simulink model "AB_Final_of_MPC_Bandwidth_Result_UnbalancedNew"  (R2022b)
settings: Solver=FixedStepDiscrete  StartTime=0.0  StopTime=Inf  FixedStep=100e-6  RelTol=1e-3  EnableMultiTasking=on
undefined symbols (not defined in the file): C28x, CPU1, CPU2, CurrentBypassValue, DiscIntNeverNeededParam, Down, GPTRIP1SEL, TZ1, Up
libraries: c2802xlib x20, simulink x17, dspstat3 x13, eeGeneralControl x10, c2837xDlib x5, c280xlib x5, PID_Lib x4, c2000lib x1, spsAlphaBetaZerotoabcLib x1
(part 9 of 10)

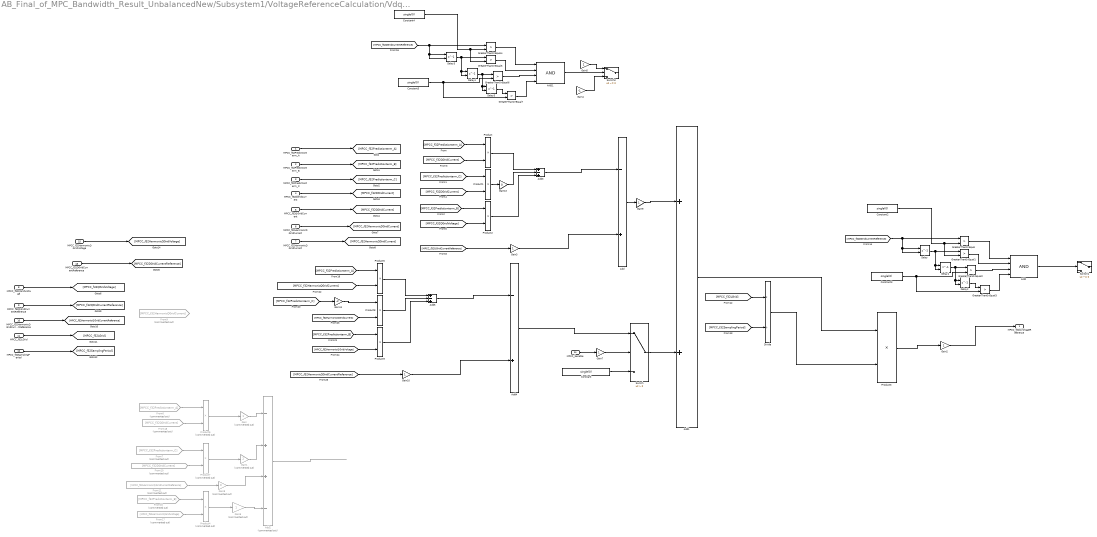
== system AB_Final_of_MPC_Bandwidth_Result_UnbalancedNew/Subsystem1/VoltageReferenceCalculation/VdqVoltageReferenceCalculation/VqVoltageReferenceCalculation ==
  MPCC_f32Predictionterm_A : Inport
  MPCC_f32Predictionterm_B : Inport  Port=2
  MPCC_f32Predictionterm_C : Inport  Port=3
  MPCC_f32DGridCurrent : Inport  Port=4
  MPCC_f32QGridCurrent : Inport  Port=5
  MPCC_f32HarmonicDGridCurrent : Inport  Port=6
  MPCC_f32HarmonicQGridCurrent : Inport  Port=7
  MPCC_f32QGridVoltage : Inport  Port=8
  MPCC_f32QGridCurrentReference : Inport  Port=9
  MPCC_f32HarmonicQGridCurrentReference : Inport  Port=10
  MPCC_f32LGrid : Inport  Port=11
  MPCC_f32SamplingPeriod : Inport  Port=12
  MPCC_f32DGridCurrentReference : Inport  Port=13
  MPCC_benable : Inport  Port=14
  MPCC_f32HarmonicQGridVoltage : Inport  Port=15
  AND : Logic  Inputs=4  AllPortsSameDT=off  OutDataTypeStr=boolean
  AND1 : Logic  Inputs=4  AllPortsSameDT=off  OutDataTypeStr=boolean
  Add : Sum  Inputs=-+
  Add1 : Sum
  Add2 : Sum  Commented=on  Inputs=-++-
  Add3 : Sum  Inputs=+-+
  Add4 : Sum  Inputs=-+
  Add5 : Sum  Inputs=+-+
  Constant{,2..5} (5 alike) : Constant  Value=single(0)
  Delay{,1..5} (6 alike) : Delay  DelayLength=1  InitialConditionSource=Input port
      settings: InputPortMap=u0,p4
  Divide : Product  Inputs=*/  RndMeth=Zero  SaturateOnIntegerOverflow=on
  From10 : From  Commented=on  GotoTag=MPCC_f32DGridCurrent
  From11 : From  Commented=on  GotoTag=MPCC_f32HarmonicQGridCurrentReference
  From15 : From  Commented=on  GotoTag=MPCC_f32Predictionterm_B
  From17 : From  Commented=on  GotoTag=MPCC_f32HarmonicQGridVoltage
  From18 : From  Commented=on  GotoTag=MPCC_f32QGridCurrent
  From6 : From  Commented=on  GotoTag=MPCC_f32Predictionterm_A
  From7 : From  Commented=on  GotoTag=MPCC_f32Predictionterm_C
  From9 : From  Commented=on  GotoTag=MPCC_f32HarmonicQGridCurrent
  Gain : Gain  Commented=on
  Gain1 : Gain  Commented=on  Gain=2
  Gain{2..3,5,7,9..10} (6 alike) : Gain
  Gain11 : Gain  Gain=-2
  Gain13 : Gain  Gain=0
  Gain4 : Gain  Gain=-1
  Gain6 : Gain  Commented=on
  Gain8 : Gain  Commented=on  Gain=0
  GreaterThanOrEqual{,1..7} (8 alike) : RelationalOperator  Operator=>  OutDataTypeStr=boolean  RndMeth=Simplest  InputSameDT=off
  Product{,1..3,5,8..9} (7 alike) : Product
  Product4 : Product  Commented=on
  Product6 : Product  Commented=on
  Product7 : Product  Commented=on
  Switch : Switch  Criteria=u2 > Threshold  SaturateOnIntegerOverflow=off  InputSameDT=off
  Switch1 : Switch  Criteria=u2 ~= 0  SaturateOnIntegerOverflow=off  InputSameDT=off
  Switch2 : Switch  Criteria=u2 ~= 0  SaturateOnIntegerOverflow=off  InputSameDT=off
  MPCC_f32QVoltageReference : Outport
  wires:
  [MPCC_f32DGridCurrent] -> Product1/2
  [MPCC_f32Predictionterm_A] -> Product/1
  [MPCC_f32QGridVoltage] -> Product2/2
  [MPCC_f32QGridCurrent] -> Product/2
  [MPCC_f32Predictionterm_C] -> Product1/1
  [MPCC_f32Predictionterm_B] -> Product2/1
  MPCC_f32Predictionterm_A/1 -> [MPCC_f32Predictionterm_A]
  MPCC_f32Predictionterm_B/1 -> [MPCC_f32Predictionterm_B]
  MPCC_f32Predictionterm_C/1 -> [MPCC_f32Predictionterm_C]
  MPCC_f32DGridCurrent/1 -> [MPCC_f32DGridCurrent]
  MPCC_f32QGridCurrent/1 -> [MPCC_f32QGridCurrent]
  MPCC_f32HarmonicDGridCurrent/1 -> [MPCC_f32HarmonicDGridCurrent]
  MPCC_f32HarmonicQGridCurrent/1 -> [MPCC_f32HarmonicQGridCurrent]
  MPCC_f32QGridVoltage/1 -> [MPCC_f32QGridVoltage]
  Constant/1 -> Switch/3
  MPCC_benable/1 -> Gain7/1
  Switch/1 -> Add1/2
  Add/1 -> Gain9/1
  MPCC_f32QGridCurrentReference/1 -> [MPCC_f32QGridCurrentReference]
  MPCC_f32HarmonicQGridCurrentReference/1 -> [MPCC_f32HarmonicQGridCurrentReference]
  [MPCC_f32QGridCurrentReference] -> Gain3/1
  MPCC_f32LGrid/1 -> [MPCC_f32LGrid]
  MPCC_f32SamplingPeriod/1 -> [MPCC_f32SamplingPeriod]
  [MPCC_f32LGrid] -> Divide/1
  [MPCC_f32SamplingPeriod] -> Divide/2
  MPCC_f32DGridCurrentReference/1 -> [MPCC_f32DGridCurrentReference]
  Gain2/1 -> MPCC_f32QVoltageReference/1
  GreaterThanOrEqual2/1 -> AND/3
  Constant3/1 -> GreaterThanOrEqual3/2, GreaterThanOrEqual2/2
  Constant2/1 -> GreaterThanOrEqual1/2, GreaterThanOrEqual/2
  Delay2/1 -> GreaterThanOrEqual3/1
  GreaterThanOrEqual1/1 -> AND/2
  Delay/1 -> GreaterThanOrEqual1/1, Delay1/2, Delay1/1
  Divide/1 -> Product3/2
  GreaterThanOrEqual/1 -> AND/1
  GreaterThanOrEqual3/1 -> AND/4
  Delay1/1 -> Delay2/2, Delay2/1, GreaterThanOrEqual2/1
  [MPCC_f32DGridCurrentReference] -> GreaterThanOrEqual/1, Delay/2, Delay/1
  Product3/1 -> Gain2/1
  AND/1 -> Switch1/2
  Product/1 -> Add3/1
  Product1/1 -> Gain13/1
  Product2/1 -> Add3/3
  Gain3/1 -> Add/2
  AND1/1 -> Switch2/2
  GreaterThanOrEqual7/1 -> AND1/4
  GreaterThanOrEqual6/1 -> AND1/3
  Delay5/1 -> GreaterThanOrEqual7/1
  GreaterThanOrEqual4/1 -> AND1/1
  Delay3/1 -> GreaterThanOrEqual5/1, Delay4/2, Delay4/1
  GreaterThanOrEqual5/1 -> AND1/2
  Constant5/1 -> GreaterThanOrEqual7/2, GreaterThanOrEqual6/2
  Delay4/1 -> Delay5/2, Delay5/1, GreaterThanOrEqual6/1
  Constant4/1 -> GreaterThanOrEqual5/2, GreaterThanOrEqual4/2
  [MPCC_f32DGridCurrentReference] -> GreaterThanOrEqual4/1, Delay3/2, Delay3/1
  Gain5/1 -> Switch2/1
  Gain4/1 -> Switch2/3
  Add1/1 -> Product3/1
  Add3/1 -> Add/1
  MPCC_f32HarmonicQGridVoltage/1 -> [MPCC_f32HarmonicQGridVoltage]
  Gain7/1 -> Switch/2
  Gain9/1 -> Add1/1
  Gain/1 -> Add2/1
  From6/1 -> Product6/1
  From11/1 -> Gain8/1
  From18/1 -> Product6/2
  From10/1 -> Product7/2
  Product7/1 -> Gain1/1
  Gain6/1 -> Add2/4
  Product6/1 -> Gain/1
  Add2/1 -> ?
  Product4/1 -> Gain6/1
  From15/1 -> Product4/1
  Gain8/1 -> Add2/3
  From7/1 -> Product7/1
  Gain1/1 -> Add2/2
  From17/1 -> Product4/2
  [MPCC_f32Predictionterm_B] -> Product9/1
  [MPCC_f32Predictionterm_C] -> Gain11/1
  [MPCC_f32HarmonicDGridCurrent] -> Product8/2
  [MPCC_f32HarmonicQGridCurrentReference] -> Gain10/1
  Add5/1 -> Add4/1
  Product5/1 -> Add5/1
  [MPCC_f32Predictionterm_A] -> Product5/1
  Gain10/1 -> Add4/2
  Product8/1 -> Add5/2
  Product9/1 -> Add5/3
  [MPCC_f32HarmonicQGridVoltage] -> Product9/2
  [MPCC_f32HarmonicQGridCurrent] -> Product5/2
  Add4/1 -> Switch/1
  Gain11/1 -> Product8/1
  Gain13/1 -> Add3/2

== system AB_Final_of_MPC_Bandwidth_Result_UnbalancedNew/Subsystem3/PLL_Loop2/SOGI 1st3/Integrator ==
  In : Inport
  Delay1 : Delay  DelayLength=1
  Delay2 : Delay  DelayLength=1
  Delay3 : Delay  DelayLength=1
  Gain : Gain  Gain=100e-6/12
  Gain1 : Gain  Gain=23
  Gain2 : Gain  Gain=16
  Gain3 : Gain  Gain=5
  Sum : Sum  Inputs=|+-
  Sum1 : Sum  Inputs=|++
  Sum2 : Sum  Inputs=|++
  Out : Outport
  wires:
  Delay2/1 -> Gain2/1, Delay3/1
  Delay1/1 -> Sum2/2, Gain1/1, Delay2/1
  Delay3/1 -> Gain3/1
  Gain2/1 -> Sum/2
  Gain1/1 -> Sum/1
  Gain3/1 -> Sum1/2
  Sum/1 -> Sum1/1
  Gain/1 -> Sum2/1
  Sum2/1 -> Delay1/1
  In/1 -> Gain/1
  Sum1/1 -> Out/1

== system AB_Final_of_MPC_Bandwidth_Result_UnbalancedNew/Subsystem3/PLL_Loop2/SOGI 1st3/Integrator1 ==
  In : Inport
  Delay1 : Delay  DelayLength=1
  Delay2 : Delay  DelayLength=1
  Delay3 : Delay  DelayLength=1
  Gain : Gain  Gain=100e-6/12
  Gain1 : Gain  Gain=23
  Gain2 : Gain  Gain=16
  Gain3 : Gain  Gain=5
  Sum : Sum  Inputs=|+-
  Sum1 : Sum  Inputs=|++
  Sum2 : Sum  Inputs=|++
  Out : Outport
  wires:
  Delay2/1 -> Gain2/1, Delay3/1
  Delay1/1 -> Sum2/2, Gain1/1, Delay2/1
  Delay3/1 -> Gain3/1
  Gain2/1 -> Sum/2
  Gain1/1 -> Sum/1
  Gain3/1 -> Sum1/2
  Sum/1 -> Sum1/1
  Gain/1 -> Sum2/1
  Sum2/1 -> Delay1/1
  In/1 -> Gain/1
  Sum1/1 -> Out/1

== system AB_Final_of_MPC_Bandwidth_Result_UnbalancedNew/Subsystem3/PLL_Loop2/SOGI 1st3/Integrator2 ==
  In : Inport
  Delay1 : Delay  DelayLength=1
  Delay2 : Delay  DelayLength=1
  Delay3 : Delay  DelayLength=1
  Gain : Gain  Gain=100e-6/12
  Gain1 : Gain  Gain=23
  Gain2 : Gain  Gain=16
  Gain3 : Gain  Gain=5
  Sum : Sum  Inputs=|+-
  Sum1 : Sum  Inputs=|++
  Sum2 : Sum  Inputs=|++
  Out : Outport
  wires:
  In/1 -> Gain/1
  Delay2/1 -> Gain2/1, Delay3/1
  Delay1/1 -> Sum2/2, Gain1/1, Delay2/1
  Delay3/1 -> Gain3/1
  Gain2/1 -> Sum/2
  Gain1/1 -> Sum/1
  Gain3/1 -> Sum1/2
  Sum/1 -> Sum1/1
  Sum1/1 -> Out/1
  Gain/1 -> Sum2/1
  Sum2/1 -> Delay1/1

== system AB_Final_of_MPC_Bandwidth_Result_UnbalancedNew/Subsystem3/PLL_Loop2/SOGI 1st5/Integrator ==
  In : Inport
  Delay1 : Delay  DelayLength=1
  Delay2 : Delay  DelayLength=1
  Delay3 : Delay  DelayLength=1
  Gain : Gain  Gain=100e-6/12
  Gain1 : Gain  Gain=23
  Gain2 : Gain  Gain=16
  Gain3 : Gain  Gain=5
  Sum : Sum  Inputs=|+-
  Sum1 : Sum  Inputs=|++
  Sum2 : Sum  Inputs=|++
  Out : Outport
  wires:
  Delay2/1 -> Gain2/1, Delay3/1
  Delay1/1 -> Sum2/2, Gain1/1, Delay2/1
  Delay3/1 -> Gain3/1
  Gain2/1 -> Sum/2
  Gain1/1 -> Sum/1
  Gain3/1 -> Sum1/2
  Sum/1 -> Sum1/1
  Gain/1 -> Sum2/1
  Sum2/1 -> Delay1/1
  In/1 -> Gain/1
  Sum1/1 -> Out/1

== system AB_Final_of_MPC_Bandwidth_Result_UnbalancedNew/Subsystem3/PLL_Loop2/SOGI 1st5/Integrator1 ==
  In : Inport
  Delay1 : Delay  DelayLength=1
  Delay2 : Delay  DelayLength=1
  Delay3 : Delay  DelayLength=1
  Gain : Gain  Gain=100e-6/12
  Gain1 : Gain  Gain=23
  Gain2 : Gain  Gain=16
  Gain3 : Gain  Gain=5
  Sum : Sum  Inputs=|+-
  Sum1 : Sum  Inputs=|++
  Sum2 : Sum  Inputs=|++
  Out : Outport
  wires:
  Delay2/1 -> Gain2/1, Delay3/1
  Delay1/1 -> Sum2/2, Gain1/1, Delay2/1
  Delay3/1 -> Gain3/1
  Gain2/1 -> Sum/2
  Gain1/1 -> Sum/1
  Gain3/1 -> Sum1/2
  Sum/1 -> Sum1/1
  Gain/1 -> Sum2/1
  Sum2/1 -> Delay1/1
  In/1 -> Gain/1
  Sum1/1 -> Out/1

== system AB_Final_of_MPC_Bandwidth_Result_UnbalancedNew/Subsystem3/PLL_Loop2/SOGI 1st5/Integrator2 ==
  In : Inport
  Delay1 : Delay  DelayLength=1
  Delay2 : Delay  DelayLength=1
  Delay3 : Delay  DelayLength=1
  Gain : Gain  Gain=100e-6/12
  Gain1 : Gain  Gain=23
  Gain2 : Gain  Gain=16
  Gain3 : Gain  Gain=5
  Sum : Sum  Inputs=|+-
  Sum1 : Sum  Inputs=|++
  Sum2 : Sum  Inputs=|++
  Out : Outport
  wires:
  In/1 -> Gain/1
  Delay2/1 -> Gain2/1, Delay3/1
  Delay1/1 -> Sum2/2, Gain1/1, Delay2/1
  Delay3/1 -> Gain3/1
  Gain2/1 -> Sum/2
  Gain1/1 -> Sum/1
  Gain3/1 -> Sum1/2
  Sum/1 -> Sum1/1
  Sum1/1 -> Out/1
  Gain/1 -> Sum2/1
  Sum2/1 -> Delay1/1

== system AB_Final_of_MPC_Bandwidth_Result_UnbalancedNew/Subsystem1/AlphaBetaDutiesCalculation/DutiesCalculation/Duty_Sector1/DutyA_Sector1 ==
  MPCC_f32AlphaVoltageReference : Inport
  MPCC_f32BetaVoltageReference : Inport  Port=2
  MPCC_f32AlphaConvVoltage1 : Inport  Port=3
  MPCC_f32AlphaConvVoltage2 : Inport  Port=4
  MPCC_f32BetaConvVoltage1 : Inport  Port=5
  MPCC_f32BetaConvVoltage2 : Inport  Port=6
  Add : Sum  Inputs=+-
  Add1 : Sum  Inputs=+-
  Data Type Conversion : DataTypeConversion  OutDataTypeStr=single  SaturateOnIntegerOverflow=off  RndMeth=Floor
  Divide : Product  Inputs=*/  RndMeth=Zero  SaturateOnIntegerOverflow=on
  Product{,1..3} (4 alike) : Product
  MPCC_f32DutyA_Sector1 : Outport
  wires:
  [MPCC_f32AlphaVoltageReference] -> Product1/1
  Divide/1 -> Data Type Conversion/1
  [MPCC_f32AlphaConvVoltage2] -> Product/2
  [MPCC_f32AlphaConvVoltage1] -> Product3/1
  Add/1 -> Divide/1
  [MPCC_f32BetaConvVoltage2] -> Product1/2
  Product/1 -> Add/1
  Add1/1 -> Divide/2
  Product2/1 -> Add1/1
  [MPCC_f32BetaConvVoltage1] -> Product2/2
  [MPCC_f32AlphaConvVoltage2] -> Product2/1
  Product3/1 -> Add1/2
  [MPCC_f32BetaConvVoltage2] -> Product3/2
  Product1/1 -> Add/2
  MPCC_f32BetaConvVoltage1/1 -> [MPCC_f32BetaConvVoltage1]
  MPCC_f32AlphaVoltageReference/1 -> [MPCC_f32AlphaVoltageReference]
  MPCC_f32AlphaConvVoltage2/1 -> [MPCC_f32AlphaConvVoltage2]
  MPCC_f32BetaVoltageReference/1 -> [MPCC_f32BetaVoltageReference]
  MPCC_f32AlphaConvVoltage1/1 -> [MPCC_f32AlphaConvVoltage1]
  MPCC_f32BetaConvVoltage2/1 -> [MPCC_f32BetaConvVoltage2]
  Data Type Conversion/1 -> MPCC_f32DutyA_Sector1/1
  [MPCC_f32BetaVoltageReference] -> Product/1

== system AB_Final_of_MPC_Bandwidth_Result_UnbalancedNew/Subsystem1/AlphaBetaDutiesCalculation/DutiesCalculation/Duty_Sector1/DutyB_Sector1 ==
  MPCC_f32AlphaVoltageReference : Inport
  MPCC_f32BetaVoltageReference : Inport  Port=2
  MPCC_f32AlphaConvVoltage1 : Inport  Port=3
  MPCC_f32AlphaConvVoltage2 : Inport  Port=4
  MPCC_f32BetaConvVoltage1 : Inport  Port=5
  MPCC_f32BetaConvVoltage2 : Inport  Port=6
  Add : Sum  Inputs=+-
  Add1 : Sum  Inputs=+-
  Data Type Conversion : DataTypeConversion  OutDataTypeStr=single  SaturateOnIntegerOverflow=off  RndMeth=Floor
  Divide : Product  Inputs=*/  RndMeth=Zero  SaturateOnIntegerOverflow=on
  Product{,1..3} (4 alike) : Product
  MPCC_f32DutyB_Sector1 : Outport
  wires:
  [MPCC_f32BetaVoltageReference] -> Product/1
  [MPCC_f32AlphaVoltageReference] -> Product1/1
  Divide/1 -> Data Type Conversion/1
  [MPCC_f32AlphaConvVoltage1] -> Product/2
  [MPCC_f32AlphaConvVoltage2] -> Product3/1
  Add/1 -> Divide/1
  [MPCC_f32BetaConvVoltage1] -> Product1/2
  Product/1 -> Add/1
  Add1/1 -> Divide/2
  Product2/1 -> Add1/1
  [MPCC_f32BetaConvVoltage2] -> Product2/2
  [MPCC_f32AlphaConvVoltage1] -> Product2/1
  Product3/1 -> Add1/2
  [MPCC_f32BetaConvVoltage1] -> Product3/2
  Product1/1 -> Add/2
  MPCC_f32BetaConvVoltage1/1 -> [MPCC_f32BetaConvVoltage1]
  MPCC_f32AlphaVoltageReference/1 -> [MPCC_f32AlphaVoltageReference]
  MPCC_f32AlphaConvVoltage2/1 -> [MPCC_f32AlphaConvVoltage2]
  MPCC_f32BetaVoltageReference/1 -> [MPCC_f32BetaVoltageReference]
  MPCC_f32AlphaConvVoltage1/1 -> [MPCC_f32AlphaConvVoltage1]
  MPCC_f32BetaConvVoltage2/1 -> [MPCC_f32BetaConvVoltage2]
  Data Type Conversion/1 -> MPCC_f32DutyB_Sector1/1

== system AB_Final_of_MPC_Bandwidth_Result_UnbalancedNew/Subsystem1/AlphaBetaDutiesCalculation/DutiesCalculation/Duty_Sector2/DutyA_Sector2 ==
  MPCC_f32AlphaVoltageReference : Inport
  MPCC_f32BetaVoltageReference : Inport  Port=2
  MPCC_f32AlphaConvVoltage2 : Inport  Port=3
  MPCC_f32AlphaConvVoltage3 : Inport  Port=4
  MPCC_f32BetaConvVoltage2 : Inport  Port=5
  MPCC_f32BetaConvVoltage3 : Inport  Port=6
  Add : Sum  Inputs=+-
  Add1 : Sum  Inputs=+-
  Data Type Conversion : DataTypeConversion  OutDataTypeStr=single  SaturateOnIntegerOverflow=off  RndMeth=Floor
  Divide : Product  Inputs=*/  RndMeth=Zero  SaturateOnIntegerOverflow=on
  Product{,1..3} (4 alike) : Product
  MPCC_f32DutyA_Sector2 : Outport
  wires:
  [MPCC_f32BetaVoltageReference] -> Product/1
  [MPCC_f32AlphaVoltageReference] -> Product1/1
  Divide/1 -> Data Type Conversion/1
  [MPCC_f32AlphaConvVoltage3] -> Product/2
  [MPCC_f32AlphaConvVoltage2] -> Product3/1
  Add/1 -> Divide/1
  [MPCC_f32BetaConvVoltage3] -> Product1/2
  Product/1 -> Add/1
  Add1/1 -> Divide/2
  Product2/1 -> Add1/1
  [MPCC_f32BetaConvVoltage2] -> Product2/2
  [MPCC_f32AlphaConvVoltage3] -> Product2/1
  Product3/1 -> Add1/2
  [MPCC_f32BetaConvVoltage3] -> Product3/2
  Product1/1 -> Add/2
  MPCC_f32BetaConvVoltage2/1 -> [MPCC_f32BetaConvVoltage2]
  MPCC_f32AlphaVoltageReference/1 -> [MPCC_f32AlphaVoltageReference]
  MPCC_f32AlphaConvVoltage3/1 -> [MPCC_f32AlphaConvVoltage3]
  MPCC_f32BetaVoltageReference/1 -> [MPCC_f32BetaVoltageReference]
  MPCC_f32AlphaConvVoltage2/1 -> [MPCC_f32AlphaConvVoltage2]
  MPCC_f32BetaConvVoltage3/1 -> [MPCC_f32BetaConvVoltage3]
  Data Type Conversion/1 -> MPCC_f32DutyA_Sector2/1

== system AB_Final_of_MPC_Bandwidth_Result_UnbalancedNew/Subsystem1/AlphaBetaDutiesCalculation/DutiesCalculation/Duty_Sector2/DutyB_Sector2 ==
  MPCC_f32AlphaVoltageReference : Inport
  MPCC_f32BetaVoltageReference : Inport  Port=2
  MPCC_f32AlphaConvVoltage2 : Inport  Port=3
  MPCC_f32AlphaConvVoltage3 : Inport  Port=4
  MPCC_f32BetaConvVoltage2 : Inport  Port=5
  MPCC_f32BetaConvVoltage3 : Inport  Port=6
  Add : Sum  Inputs=+-
  Add1 : Sum  Inputs=+-
  Data Type Conversion : DataTypeConversion  OutDataTypeStr=single  SaturateOnIntegerOverflow=off  RndMeth=Floor
  Divide : Product  Inputs=*/  RndMeth=Zero  SaturateOnIntegerOverflow=on
  Product{,1..3} (4 alike) : Product
  MPCC_f32DutyB_Sector2 : Outport
  wires:
  [MPCC_f32BetaVoltageReference] -> Product/1
  [MPCC_f32AlphaVoltageReference] -> Product1/1
  Divide/1 -> Data Type Conversion/1
  [MPCC_f32AlphaConvVoltage2] -> Product/2
  [MPCC_f32AlphaConvVoltage3] -> Product3/1
  Add/1 -> Divide/1
  [MPCC_f32BetaConvVoltage2] -> Product1/2
  Product/1 -> Add/1
  Add1/1 -> Divide/2
  Product2/1 -> Add1/1
  [MPCC_f32BetaConvVoltage3] -> Product2/2
  [MPCC_f32AlphaConvVoltage2] -> Product2/1
  Product3/1 -> Add1/2
  [MPCC_f32BetaConvVoltage2] -> Product3/2
  Product1/1 -> Add/2
  MPCC_f32AlphaVoltageReference/1 -> [MPCC_f32AlphaVoltageReference]
  MPCC_f32BetaVoltageReference/1 -> [MPCC_f32BetaVoltageReference]
  MPCC_f32AlphaConvVoltage3/1 -> [MPCC_f32AlphaConvVoltage3]
  MPCC_f32BetaConvVoltage2/1 -> [MPCC_f32BetaConvVoltage2]
  MPCC_f32AlphaConvVoltage2/1 -> [MPCC_f32AlphaConvVoltage2]
  MPCC_f32BetaConvVoltage3/1 -> [MPCC_f32BetaConvVoltage3]
  Data Type Conversion/1 -> MPCC_f32DutyB_Sector2/1

== system AB_Final_of_MPC_Bandwidth_Result_UnbalancedNew/Subsystem1/AlphaBetaDutiesCalculation/DutiesCalculation/Duty_Sector3/DutyA_Sector3 ==
  MPCC_f32AlphaVoltageReference : Inport
  MPCC_f32BetaVoltageReference : Inport  Port=2
  MPCC_f32AlphaConvVoltage3 : Inport  Port=3
  MPCC_f32AlphaConvVoltage4 : Inport  Port=4
  MPCC_f32BetaConvVoltage3 : Inport  Port=5
  MPCC_f32BetaConvVoltage4 : Inport  Port=6
  Add : Sum  Inputs=+-
  Add1 : Sum  Inputs=+-
  Data Type Conversion : DataTypeConversion  OutDataTypeStr=single  SaturateOnIntegerOverflow=off  RndMeth=Floor
  Divide : Product  Inputs=*/  RndMeth=Zero  SaturateOnIntegerOverflow=on
  Product{,1..3} (4 alike) : Product
  MPCC_f32DutyA_Sector3 : Outport
  wires:
  [MPCC_f32BetaVoltageReference] -> Product/1
  [MPCC_f32AlphaVoltageReference] -> Product1/1
  Divide/1 -> Data Type Conversion/1
  [MPCC_f32AlphaConvVoltage4] -> Product/2
  [MPCC_f32AlphaConvVoltage3] -> Product3/1
  Add/1 -> Divide/1
  [MPCC_f32BetaConvVoltage4] -> Product1/2
  Product/1 -> Add/1
  Add1/1 -> Divide/2
  Product2/1 -> Add1/1
  [MPCC_f32BetaConvVoltage3] -> Product2/2
  [MPCC_f32AlphaConvVoltage4] -> Product2/1
  Product3/1 -> Add1/2
  [MPCC_f32BetaConvVoltage4] -> Product3/2
  Product1/1 -> Add/2
  MPCC_f32BetaConvVoltage3/1 -> [MPCC_f32BetaConvVoltage3]
  MPCC_f32AlphaVoltageReference/1 -> [MPCC_f32AlphaVoltageReference]
  MPCC_f32AlphaConvVoltage4/1 -> [MPCC_f32AlphaConvVoltage4]
  MPCC_f32BetaVoltageReference/1 -> [MPCC_f32BetaVoltageReference]
  MPCC_f32AlphaConvVoltage3/1 -> [MPCC_f32AlphaConvVoltage3]
  MPCC_f32BetaConvVoltage4/1 -> [MPCC_f32BetaConvVoltage4]
  Data Type Conversion/1 -> MPCC_f32DutyA_Sector3/1

== system AB_Final_of_MPC_Bandwidth_Result_UnbalancedNew/Subsystem1/AlphaBetaDutiesCalculation/DutiesCalculation/Duty_Sector3/DutyB_Sector3 ==
  MPCC_f32AlphaVoltageReference : Inport
  MPCC_f32BetaVoltageReference : Inport  Port=2
  MPCC_f32AlphaConvVoltage3 : Inport  Port=3
  MPCC_f32AlphaConvVoltage4 : Inport  Port=4
  MPCC_f32BetaConvVoltage3 : Inport  Port=5
  MPCC_f32BetaConvVoltage4 : Inport  Port=6
  Add : Sum  Inputs=+-
  Add1 : Sum  Inputs=+-
  Data Type Conversion : DataTypeConversion  OutDataTypeStr=single  SaturateOnIntegerOverflow=off  RndMeth=Floor
  Divide : Product  Inputs=*/  RndMeth=Zero  SaturateOnIntegerOverflow=on
  Product{,1..3} (4 alike) : Product
  MPCC_f32DutyB_Sector3 : Outport
  wires:
  [MPCC_f32BetaVoltageReference] -> Product/1
  [MPCC_f32AlphaVoltageReference] -> Product1/1
  Divide/1 -> Data Type Conversion/1
  [MPCC_f32AlphaConvVoltage3] -> Product/2
  [MPCC_f32AlphaConvVoltage4] -> Product3/1
  Add/1 -> Divide/1
  [MPCC_f32BetaConvVoltage3] -> Product1/2
  Product/1 -> Add/1
  Add1/1 -> Divide/2
  Product2/1 -> Add1/1
  [MPCC_f32BetaConvVoltage4] -> Product2/2
  [MPCC_f32AlphaConvVoltage3] -> Product2/1
  Product3/1 -> Add1/2
  [MPCC_f32BetaConvVoltage3] -> Product3/2
  Product1/1 -> Add/2
  MPCC_f32BetaVoltageReference/1 -> [MPCC_f32BetaVoltageReference]
  MPCC_f32AlphaConvVoltage3/1 -> [MPCC_f32AlphaConvVoltage3]
  MPCC_f32AlphaConvVoltage4/1 -> [MPCC_f32AlphaConvVoltage4]
  MPCC_f32AlphaVoltageReference/1 -> [MPCC_f32AlphaVoltageReference]
  MPCC_f32BetaConvVoltage4/1 -> [MPCC_f32BetaConvVoltage4]
  MPCC_f32BetaConvVoltage3/1 -> [MPCC_f32BetaConvVoltage3]
  Data Type Conversion/1 -> MPCC_f32DutyB_Sector3/1

== system AB_Final_of_MPC_Bandwidth_Result_UnbalancedNew/Subsystem1/AlphaBetaDutiesCalculation/DutiesCalculation/Duty_Sector4/DutyA_Sector4 ==
  MPCC_f32AlphaVoltageReference : Inport
  MPCC_f32BetaVoltageReference : Inport  Port=2
  MPCC_f32AlphaConvVoltage4 : Inport  Port=3
  MPCC_f32AlphaConvVoltage5 : Inport  Port=4
  MPCC_f32BetaConvVoltage4 : Inport  Port=5
  MPCC_f32BetaConvVoltage5 : Inport  Port=6
  Add : Sum  Inputs=+-
  Add1 : Sum  Inputs=+-
  Data Type Conversion : DataTypeConversion  OutDataTypeStr=single  SaturateOnIntegerOverflow=off  RndMeth=Floor
  Divide : Product  Inputs=*/  RndMeth=Zero  SaturateOnIntegerOverflow=on
  Product{,1..3} (4 alike) : Product
  MPCC_f32DutyA_Sector4 : Outport
  wires:
  [MPCC_f32BetaVoltageReference] -> Product/1
  [MPCC_f32AlphaVoltageReference] -> Product1/1
  Divide/1 -> Data Type Conversion/1
  [MPCC_f32AlphaConvVoltage5] -> Product/2
  [MPCC_f32AlphaConvVoltage4] -> Product3/1
  Add/1 -> Divide/1
  [MPCC_f32BetaConvVoltage5] -> Product1/2
  Product/1 -> Add/1
  Add1/1 -> Divide/2
  Product2/1 -> Add1/1
  [MPCC_f32BetaConvVoltage4] -> Product2/2
  [MPCC_f32AlphaConvVoltage5] -> Product2/1
  Product3/1 -> Add1/2
  [MPCC_f32BetaConvVoltage5] -> Product3/2
  Product1/1 -> Add/2
  MPCC_f32BetaConvVoltage4/1 -> [MPCC_f32BetaConvVoltage4]
  MPCC_f32AlphaVoltageReference/1 -> [MPCC_f32AlphaVoltageReference]
  MPCC_f32AlphaConvVoltage5/1 -> [MPCC_f32AlphaConvVoltage5]
  MPCC_f32BetaVoltageReference/1 -> [MPCC_f32BetaVoltageReference]
  MPCC_f32AlphaConvVoltage4/1 -> [MPCC_f32AlphaConvVoltage4]
  MPCC_f32BetaConvVoltage5/1 -> [MPCC_f32BetaConvVoltage5]
  Data Type Conversion/1 -> MPCC_f32DutyA_Sector4/1

== system AB_Final_of_MPC_Bandwidth_Result_UnbalancedNew/Subsystem1/AlphaBetaDutiesCalculation/DutiesCalculation/Duty_Sector4/DutyB_Sector4 ==
  MPCC_f32AlphaVoltageReference : Inport
  MPCC_f32BetaVoltageReference : Inport  Port=2
  MPCC_f32AlphaConvVoltage4 : Inport  Port=3
  MPCC_f32AlphaConvVoltage5 : Inport  Port=4
  MPCC_f32BetaConvVoltage4 : Inport  Port=5
  MPCC_f32BetaConvVoltage5 : Inport  Port=6
  Add : Sum  Inputs=+-
  Add1 : Sum  Inputs=+-
  Data Type Conversion : DataTypeConversion  OutDataTypeStr=single  SaturateOnIntegerOverflow=off  RndMeth=Floor
  Divide : Product  Inputs=*/  RndMeth=Zero  SaturateOnIntegerOverflow=on
  Product{,1..3} (4 alike) : Product
  MPCC_f32DutyB_Sector4 : Outport
  wires:
  [MPCC_f32BetaVoltageReference] -> Product/1
  [MPCC_f32AlphaVoltageReference] -> Product1/1
  Divide/1 -> Data Type Conversion/1
  [MPCC_f32AlphaConvVoltage4] -> Product/2
  [MPCC_f32AlphaConvVoltage5] -> Product3/1
  Add/1 -> Divide/1
  [MPCC_f32BetaConvVoltage4] -> Product1/2
  Product/1 -> Add/1
  Add1/1 -> Divide/2
  Product2/1 -> Add1/1
  [MPCC_f32BetaConvVoltage5] -> Product2/2
  [MPCC_f32AlphaConvVoltage4] -> Product2/1
  Product3/1 -> Add1/2
  [MPCC_f32BetaConvVoltage4] -> Product3/2
  Product1/1 -> Add/2
  MPCC_f32AlphaVoltageReference/1 -> [MPCC_f32AlphaVoltageReference]
  MPCC_f32BetaVoltageReference/1 -> [MPCC_f32BetaVoltageReference]
  MPCC_f32BetaConvVoltage5/1 -> [MPCC_f32BetaConvVoltage5]
  MPCC_f32BetaConvVoltage4/1 -> [MPCC_f32BetaConvVoltage4]
  MPCC_f32AlphaConvVoltage4/1 -> [MPCC_f32AlphaConvVoltage4]
  MPCC_f32AlphaConvVoltage5/1 -> [MPCC_f32AlphaConvVoltage5]
  Data Type Conversion/1 -> MPCC_f32DutyB_Sector4/1

== system AB_Final_of_MPC_Bandwidth_Result_UnbalancedNew/Subsystem1/AlphaBetaDutiesCalculation/DutiesCalculation/Duty_Sector5/DutyA_Sector5 ==
  MPCC_f32AlphaVoltageReference : Inport
  MPCC_f32BetaVoltageReference : Inport  Port=2
  MPCC_f32AlphaConvVoltage5 : Inport  Port=3
  MPCC_f32AlphaConvVoltage6 : Inport  Port=4
  MPCC_f32BetaConvVoltage5 : Inport  Port=5
  MPCC_f32BetaConvVoltage6 : Inport  Port=6
  Add : Sum  Inputs=+-
  Add1 : Sum  Inputs=+-
  Data Type Conversion : DataTypeConversion  OutDataTypeStr=single  SaturateOnIntegerOverflow=off  RndMeth=Floor
  Divide : Product  Inputs=*/  RndMeth=Zero  SaturateOnIntegerOverflow=on
  Product{,1..3} (4 alike) : Product
  MPCC_f32DutyA_Sector5 : Outport
  wires:
  [MPCC_f32BetaVoltageReference] -> Product/1
  [MPCC_f32AlphaVoltageReference] -> Product1/1
  Divide/1 -> Data Type Conversion/1
  [MPCC_f32AlphaConvVoltage6] -> Product/2
  [MPCC_f32AlphaConvVoltage5] -> Product3/1
  Add/1 -> Divide/1
  [MPCC_f32BetaConvVoltage6] -> Product1/2
  Product/1 -> Add/1
  Add1/1 -> Divide/2
  Product2/1 -> Add1/1
  [MPCC_f32BetaConvVoltage5] -> Product2/2
  [MPCC_f32AlphaConvVoltage6] -> Product2/1
  Product3/1 -> Add1/2
  [MPCC_f32BetaConvVoltage6] -> Product3/2
  Product1/1 -> Add/2
  MPCC_f32BetaConvVoltage5/1 -> [MPCC_f32BetaConvVoltage5]
  MPCC_f32AlphaVoltageReference/1 -> [MPCC_f32AlphaVoltageReference]
  MPCC_f32AlphaConvVoltage6/1 -> [MPCC_f32AlphaConvVoltage6]
  MPCC_f32BetaVoltageReference/1 -> [MPCC_f32BetaVoltageReference]
  MPCC_f32AlphaConvVoltage5/1 -> [MPCC_f32AlphaConvVoltage5]
  MPCC_f32BetaConvVoltage6/1 -> [MPCC_f32BetaConvVoltage6]
  Data Type Conversion/1 -> MPCC_f32DutyA_Sector5/1

== system AB_Final_of_MPC_Bandwidth_Result_UnbalancedNew/Subsystem1/AlphaBetaDutiesCalculation/DutiesCalculation/Duty_Sector5/DutyB_Sector5 ==
  MPCC_f32AlphaVoltageReference : Inport
  MPCC_f32BetaVoltageReference : Inport  Port=2
  MPCC_f32AlphaConvVoltage5 : Inport  Port=3
  MPCC_f32AlphaConvVoltage6 : Inport  Port=4
  MPCC_f32BetaConvVoltage5 : Inport  Port=5
  MPCC_f32BetaConvVoltage6 : Inport  Port=6
  Add : Sum  Inputs=+-
  Add1 : Sum  Inputs=+-
  Data Type Conversion : DataTypeConversion  OutDataTypeStr=single  SaturateOnIntegerOverflow=off  RndMeth=Floor
  Divide : Product  Inputs=*/  RndMeth=Zero  SaturateOnIntegerOverflow=on
  Product{,1..3} (4 alike) : Product
  MPCC_f32DutyB_Sector5 : Outport
  wires:
  [MPCC_f32BetaVoltageReference] -> Product/1
  [MPCC_f32AlphaVoltageReference] -> Product1/1
  Divide/1 -> Data Type Conversion/1
  [MPCC_f32AlphaConvVoltage5] -> Product/2
  [MPCC_f32AlphaConvVoltage6] -> Product3/1
  Add/1 -> Divide/1
  [MPCC_f32BetaConvVoltage5] -> Product1/2
  Product/1 -> Add/1
  Add1/1 -> Divide/2
  Product2/1 -> Add1/1
  [MPCC_f32BetaConvVoltage6] -> Product2/2
  [MPCC_f32AlphaConvVoltage5] -> Product2/1
  Product3/1 -> Add1/2
  [MPCC_f32BetaConvVoltage5] -> Product3/2
  Product1/1 -> Add/2
  MPCC_f32BetaConvVoltage6/1 -> [MPCC_f32BetaConvVoltage6]
  MPCC_f32BetaConvVoltage5/1 -> [MPCC_f32BetaConvVoltage5]
  MPCC_f32BetaVoltageReference/1 -> [MPCC_f32BetaVoltageReference]
  MPCC_f32AlphaConvVoltage5/1 -> [MPCC_f32AlphaConvVoltage5]
  MPCC_f32AlphaConvVoltage6/1 -> [MPCC_f32AlphaConvVoltage6]
  MPCC_f32AlphaVoltageReference/1 -> [MPCC_f32AlphaVoltageReference]
  Data Type Conversion/1 -> MPCC_f32DutyB_Sector5/1

== system AB_Final_of_MPC_Bandwidth_Result_UnbalancedNew/Subsystem1/AlphaBetaDutiesCalculation/DutiesCalculation/Duty_Sector6/DutyA_Sector6 ==
  MPCC_f32AlphaVoltageReference : Inport
  MPCC_f32BetaVoltageReference : Inport  Port=2
  MPCC_f32AlphaConvVoltage6 : Inport  Port=3
  MPCC_f32AlphaConvVoltage1 : Inport  Port=4
  MPCC_f32BetaConvVoltage6 : Inport  Port=5
  MPCC_f32BetaConvVoltage1 : Inport  Port=6
  Add : Sum  Inputs=+-
  Add1 : Sum  Inputs=+-
  Data Type Conversion : DataTypeConversion  OutDataTypeStr=single  SaturateOnIntegerOverflow=off  RndMeth=Floor
  Divide : Product  Inputs=*/  RndMeth=Zero  SaturateOnIntegerOverflow=on
  Product{,1..3} (4 alike) : Product
  MPCC_f32DutyA_Sector6 : Outport
  wires:
  [MPCC_f32BetaVoltageReference] -> Product/1
  [MPCC_f32AlphaVoltageReference] -> Product1/1
  Divide/1 -> Data Type Conversion/1
  [MPCC_f32AlphaConvVoltage1] -> Product/2
  [MPCC_f32AlphaConvVoltage6] -> Product3/1
  Add/1 -> Divide/1
  [MPCC_f32BetaConvVoltage1] -> Product1/2
  Product/1 -> Add/1
  Add1/1 -> Divide/2
  Product2/1 -> Add1/1
  [MPCC_f32BetaConvVoltage6] -> Product2/2
  [MPCC_f32AlphaConvVoltage1] -> Product2/1
  Product3/1 -> Add1/2
  [MPCC_f32BetaConvVoltage1] -> Product3/2
  Product1/1 -> Add/2
  MPCC_f32BetaConvVoltage6/1 -> [MPCC_f32BetaConvVoltage6]
  MPCC_f32AlphaVoltageReference/1 -> [MPCC_f32AlphaVoltageReference]
  MPCC_f32AlphaConvVoltage1/1 -> [MPCC_f32AlphaConvVoltage1]
  MPCC_f32BetaVoltageReference/1 -> [MPCC_f32BetaVoltageReference]
  MPCC_f32AlphaConvVoltage6/1 -> [MPCC_f32AlphaConvVoltage6]
  MPCC_f32BetaConvVoltage1/1 -> [MPCC_f32BetaConvVoltage1]
  Data Type Conversion/1 -> MPCC_f32DutyA_Sector6/1

== system AB_Final_of_MPC_Bandwidth_Result_UnbalancedNew/Subsystem1/AlphaBetaDutiesCalculation/DutiesCalculation/Duty_Sector6/DutyB_Sector6 ==
  MPCC_f32AlphaVoltageReference : Inport
  MPCC_f32BetaVoltageReference : Inport  Port=2
  MPCC_f32AlphaConvVoltage6 : Inport  Port=3
  MPCC_f32AlphaConvVoltage1 : Inport  Port=4
  MPCC_f32BetaConvVoltage6 : Inport  Port=5
  MPCC_f32BetaConvVoltage1 : Inport  Port=6
  Add : Sum  Inputs=+-
  Add1 : Sum  Inputs=+-
  Data Type Conversion : DataTypeConversion  OutDataTypeStr=single  SaturateOnIntegerOverflow=off  RndMeth=Floor
  Divide : Product  Inputs=*/  RndMeth=Zero  SaturateOnIntegerOverflow=on
  Product{,1..3} (4 alike) : Product
  MPCC_f32DutyB_Sector6 : Outport
  wires:
  [MPCC_f32BetaVoltageReference] -> Product/1
  [MPCC_f32AlphaVoltageReference] -> Product1/1
  Divide/1 -> Data Type Conversion/1
  [MPCC_f32AlphaConvVoltage6] -> Product/2
  [MPCC_f32AlphaConvVoltage1] -> Product3/1
  Add/1 -> Divide/1
  [MPCC_f32BetaConvVoltage6] -> Product1/2
  Product/1 -> Add/1
  Add1/1 -> Divide/2
  Product2/1 -> Add1/1
  [MPCC_f32BetaConvVoltage1] -> Product2/2
  [MPCC_f32AlphaConvVoltage6] -> Product2/1
  Product3/1 -> Add1/2
  [MPCC_f32BetaConvVoltage6] -> Product3/2
  Product1/1 -> Add/2
  MPCC_f32BetaConvVoltage1/1 -> [MPCC_f32BetaConvVoltage1]
  MPCC_f32AlphaVoltageReference/1 -> [MPCC_f32AlphaVoltageReference]
  MPCC_f32BetaVoltageReference/1 -> [MPCC_f32BetaVoltageReference]
  MPCC_f32AlphaConvVoltage6/1 -> [MPCC_f32AlphaConvVoltage6]
  MPCC_f32BetaConvVoltage6/1 -> [MPCC_f32BetaConvVoltage6]
  MPCC_f32AlphaConvVoltage1/1 -> [MPCC_f32AlphaConvVoltage1]
  Data Type Conversion/1 -> MPCC_f32DutyB_Sector6/1

== system AB_Final_of_MPC_Bandwidth_Result_UnbalancedNew/Subsystem1/GridCurrentSecondPrediction/CostFunctionofVoltageVectors/CostFunctionVoltage1/CostFunctionVoltage1 ==
  MPCC_f32DGridCurrentReference : Inport
  MPCC_f32QGridCurrentReference : Inport  Port=2
  MPCC_f32DGridCurrent_K_2_Voltage1 : Inport  Port=3
  MPCC_f32QGridCurrent_K_2_Voltage1 : Inport  Port=4
  MPCC_f32DGridCurrent : Inport  Port=5
  MPCC_f32QGridCurrent : Inport  Port=6
  MPCC_f32DGridCurrent1 : Inport  Port=7
  MPCC_f32QGridCurrent1 : Inport  Port=8
  Abs{,1..5} (6 alike) : Abs  SaturateOnIntegerOverflow=off
  Add{,2..6} (6 alike) : Sum  Inputs=+-
  Add1 : Sum  Inputs=++++++
  Constant : Constant  Value=single(0)
  Constant1 : Constant  Value=single(0)
  Gain : Gain
  Gain1 : Gain
  Gain2 : Gain  Gain=0
  Gain3 : Gain  Gain=0
  Square : Math  Operator=square
  Square1 : Math  Operator=square
  MPCC_f32CostFunction_Voltage1 : Outport
  wires:
  MPCC_f32QGridCurrentReference/1 -> [MPCC_f32QGridCurrentReference]
  MPCC_f32DGridCurrentReference/1 -> [MPCC_f32DGridCurrentReference]
  MPCC_f32QGridCurrent_K_2_Voltage1/1 -> [MPCC_f32QGridCurrent_K_2_Voltage1]
  MPCC_f32DGridCurrent_K_2_Voltage1/1 -> [MPCC_f32DGridCurrent_K_2_Voltage1]
  [MPCC_f32DGridCurrentReference] -> Add/1
  [MPCC_f32DGridCurrent_K_2_Voltage1] -> Add/2
  Add/1 -> Abs/1
  Abs/1 -> Add1/1
  Add2/1 -> Abs1/1
  [MPCC_f32QGridCurrentReference] -> Add2/1
  [MPCC_f32QGridCurrent_K_2_Voltage1] -> Add2/2
  MPCC_f32QGridCurrent/1 -> [MPCC_f32QGridCurrent]
  MPCC_f32DGridCurrent/1 -> [MPCC_f32DGridCurrent]
  [MPCC_f32QGridCurrent] -> Add4/1
  Add4/1 -> Abs3/1
  Add3/1 -> Abs2/1
  [MPCC_f32QGridCurrent_K_2_Voltage1] -> Add4/2
  [MPCC_f32DGridCurrent] -> Add3/1
  [MPCC_f32DGridCurrent_K_2_Voltage1] -> Add3/2
  Abs1/1 -> Add1/2
  Abs2/1 -> Gain/1
  Abs3/1 -> Gain1/1
  Add1/1 -> MPCC_f32CostFunction_Voltage1/1
  Gain/1 -> Add1/3
  Gain1/1 -> Add1/4
  MPCC_f32DGridCurrent1/1 -> [MPCC_f32DGridCurrent1]
  MPCC_f32QGridCurrent1/1 -> [MPCC_f32QGridCurrent1]
  Abs4/1 -> Gain2/1
  Add5/1 -> Abs4/1
  [MPCC_f32QGridCurrent1] -> Add5/2
  Constant/1 -> Add5/1
  Gain2/1 -> Add1/6
  Constant1/1 -> Add6/1
  Add6/1 -> Abs5/1
  [MPCC_f32DGridCurrent1] -> Add6/2
  Abs5/1 -> Gain3/1
  Gain3/1 -> Add1/5

== system AB_Final_of_MPC_Bandwidth_Result_UnbalancedNew/Subsystem1/GridCurrentSecondPrediction/CostFunctionofVoltageVectors/CostFunctionVoltage1/DGridCurrentSecondPrediction_Voltage1 ==
  MPCC_f32Predictionterm_A : Inport
  MPCC_f32Predictionterm_B : Inport  Port=2
  MPCC_f32Predictionterm_C : Inport  Port=3
  MPCC_f32DGridCurrent_K_1 : Inport  Port=4
  MPCC_f32QGridCurrent_K_1 : Inport  Port=5
  MPCC_f32DGridVoltage : Inport  Port=6
  MPCC_f32DVoltageVector1 : Inport  Port=7
  Add1 : Sum  Inputs=+++-
  Gain : Gain  Gain=0
  Product : Product
  Product1 : Product
  Product2 : Product  OutDataTypeStr=Inherit: Inherit via back propagation
  Product4 : Product  OutDataTypeStr=Inherit: Inherit via back propagation
  MPCC_f32DGridCurrent_K_2_Voltage1 : Outport
  wires:
  [MPCC_f32DGridCurrent_K_1] -> Product/2
  MPCC_f32Predictionterm_A/1 -> [MPCC_f32Predictionterm_A]
  [MPCC_f32DGridVoltage] -> Product2/2
  Product1/1 -> Gain/1
  [MPCC_f32Predictionterm_C] -> Product1/1
  Product/1 -> Add1/1
  [MPCC_f32DVoltageVector1] -> Product4/2
  MPCC_f32DGridVoltage/1 -> [MPCC_f32DGridVoltage]
  [MPCC_f32Predictionterm_A] -> Product/1
  [MPCC_f32Predictionterm_B] -> Product4/1
  [MPCC_f32Predictionterm_B] -> Product2/1
  [MPCC_f32QGridCurrent_K_1] -> Product1/2
  MPCC_f32DGridCurrent_K_1/1 -> [MPCC_f32DGridCurrent_K_1]
  MPCC_f32QGridCurrent_K_1/1 -> [MPCC_f32QGridCurrent_K_1]
  MPCC_f32Predictionterm_C/1 -> [MPCC_f32Predictionterm_C]
  MPCC_f32Predictionterm_B/1 -> [MPCC_f32Predictionterm_B]
  Add1/1 -> MPCC_f32DGridCurrent_K_2_Voltage1/1
  MPCC_f32DVoltageVector1/1 -> [MPCC_f32DVoltageVector1]
  Product2/1 -> Add1/3
  Product4/1 -> Add1/4
  Gain/1 -> Add1/2

== system AB_Final_of_MPC_Bandwidth_Result_UnbalancedNew/Subsystem1/GridCurrentSecondPrediction/CostFunctionofVoltageVectors/CostFunctionVoltage1/QGridCurrentSecondPrediction_Voltage1 ==
  MPCC_f32Predictionterm_A : Inport
  MPCC_f32Predictionterm_B : Inport  Port=2
  MPCC_f32Predictionterm_C : Inport  Port=3
  MPCC_f32DGridCurrent_K_1 : Inport  Port=4
  MPCC_f32QGridCurrent_K_1 : Inport  Port=5
  MPCC_f32QGridVoltage : Inport  Port=6
  MPCC_f32QVoltageVector1 : Inport  Port=7
  Add1 : Sum  Inputs=+-+-
  Gain : Gain  Gain=0
  Product : Product
  Product1 : Product
  Product2 : Product  OutDataTypeStr=Inherit: Inherit via back propagation
  Product4 : Product  OutDataTypeStr=Inherit: Inherit via back propagation
  MPCC_f32QGridCurrent_K_2_Voltage1 : Outport
  wires:
  [MPCC_f32QGridCurrent_K_1] -> Product/2
  MPCC_f32Predictionterm_A/1 -> [MPCC_f32Predictionterm_A]
  [MPCC_f32QGridVoltage] -> Product2/2
  Product1/1 -> Gain/1
  [MPCC_f32Predictionterm_C] -> Product1/1
  Product/1 -> Add1/1
  [MPCC_f32QVoltageVector1] -> Product4/2
  [MPCC_f32Predictionterm_A] -> Product/1
  [MPCC_f32Predictionterm_B] -> Product4/1
  [MPCC_f32Predictionterm_B] -> Product2/1
  [MPCC_f32DGridCurrent_K_1] -> Product1/2
  MPCC_f32DGridCurrent_K_1/1 -> [MPCC_f32DGridCurrent_K_1]
  MPCC_f32QGridCurrent_K_1/1 -> [MPCC_f32QGridCurrent_K_1]
  MPCC_f32Predictionterm_C/1 -> [MPCC_f32Predictionterm_C]
  MPCC_f32QGridVoltage/1 -> [MPCC_f32QGridVoltage]
  MPCC_f32Predictionterm_B/1 -> [MPCC_f32Predictionterm_B]
  Add1/1 -> MPCC_f32QGridCurrent_K_2_Voltage1/1
  MPCC_f32QVoltageVector1/1 -> [MPCC_f32QVoltageVector1]
  Product2/1 -> Add1/3
  Product4/1 -> Add1/4
  Gain/1 -> Add1/2

== system AB_Final_of_MPC_Bandwidth_Result_UnbalancedNew/Subsystem1/GridCurrentSecondPrediction/CostFunctionofVoltageVectors/CostFunctionVoltage2/CostFunctionVoltage2 ==
  MPCC_f32DGridCurrentReference : Inport
  MPCC_f32QGridCurrentReference : Inport  Port=2
  MPCC_f32DGridCurrent_K_2_Voltage2 : Inport  Port=3
  MPCC_f32QGridCurrent_K_2_Voltage2 : Inport  Port=4
  MPCC_f32DGridCurrent : Inport  Port=5
  MPCC_f32QGridCurrent : Inport  Port=6
  MPCC_f32DGridCurrent1 : Inport  Port=7
  MPCC_f32QGridCurrent1 : Inport  Port=8
  Abs{,1..5} (6 alike) : Abs  SaturateOnIntegerOverflow=off
  Add{,2..6} (6 alike) : Sum  Inputs=+-
  Add1 : Sum  Inputs=++++++
  Constant : Constant  Value=single(0)
  Constant1 : Constant  Value=single(0)
  Gain : Gain
  Gain1 : Gain
  Gain2 : Gain  Gain=0
  Gain3 : Gain  Gain=0
  Square : Math  Operator=square
  Square1 : Math  Operator=square
  MPCC_f32CostFunction_Voltage2 : Outport
  wires:
  MPCC_f32QGridCurrentReference/1 -> [MPCC_f32QGridCurrentReference]
  MPCC_f32DGridCurrentReference/1 -> [MPCC_f32DGridCurrentReference]
  MPCC_f32QGridCurrent_K_2_Voltage2/1 -> [MPCC_f32QGridCurrent_K_2_Voltage2]
  MPCC_f32DGridCurrent_K_2_Voltage2/1 -> [MPCC_f32DGridCurrent_K_2_Voltage2]
  [MPCC_f32DGridCurrentReference] -> Add/1
  [MPCC_f32DGridCurrent_K_2_Voltage2] -> Add/2
  [MPCC_f32QGridCurrentReference] -> Add2/1
  [MPCC_f32QGridCurrent_K_2_Voltage2] -> Add2/2
  MPCC_f32QGridCurrent/1 -> [MPCC_f32QGridCurrent]
  MPCC_f32DGridCurrent/1 -> [MPCC_f32DGridCurrent]
  [MPCC_f32QGridCurrent] -> Add4/1
  Add4/1 -> Abs3/1
  Add3/1 -> Abs2/1
  [MPCC_f32QGridCurrent_K_2_Voltage2] -> Add4/2
  [MPCC_f32DGridCurrent] -> Add3/1
  [MPCC_f32DGridCurrent_K_2_Voltage2] -> Add3/2
  Abs2/1 -> Gain/1
  Abs3/1 -> Gain1/1
  Add1/1 -> MPCC_f32CostFunction_Voltage2/1
  Gain/1 -> Add1/3
  Gain1/1 -> Add1/4
  Abs1/1 -> Add1/2
  Add2/1 -> Abs1/1
  Abs/1 -> Add1/1
  Add/1 -> Abs/1
  MPCC_f32DGridCurrent1/1 -> [MPCC_f32DGridCurrent1]
  MPCC_f32QGridCurrent1/1 -> [MPCC_f32QGridCurrent1]
  Constant/1 -> Add5/1
  Add5/1 -> Abs4/1
  Add6/1 -> Abs5/1
  Abs4/1 -> Gain2/1
  Constant1/1 -> Add6/1
  [MPCC_f32DGridCurrent1] -> Add6/2
  [MPCC_f32QGridCurrent1] -> Add5/2
  Gain2/1 -> Add1/6
  Abs5/1 -> Gain3/1
  Gain3/1 -> Add1/5

== system AB_Final_of_MPC_Bandwidth_Result_UnbalancedNew/Subsystem1/GridCurrentSecondPrediction/CostFunctionofVoltageVectors/CostFunctionVoltage2/DGridCurrentSecondPrediction_Voltage2 ==
  MPCC_f32Predictionterm_A : Inport
  MPCC_f32Predictionterm_B : Inport  Port=2
  MPCC_f32Predictionterm_C : Inport  Port=3
  MPCC_f32DGridCurrent_K_1 : Inport  Port=4
  MPCC_f32QGridCurrent_K_1 : Inport  Port=5
  MPCC_f32DGridVoltage : Inport  Port=6
  MPCC_f32DVoltageVector2 : Inport  Port=7
  Add1 : Sum  Inputs=+++-
  Gain : Gain  Gain=0
  Product : Product
  Product1 : Product
  Product2 : Product  OutDataTypeStr=Inherit: Inherit via back propagation
  Product4 : Product  OutDataTypeStr=Inherit: Inherit via back propagation
  MPCC_f32DGridCurrent_K_2_Voltage2 : Outport
  wires:
  [MPCC_f32DGridCurrent_K_1] -> Product/2
  MPCC_f32Predictionterm_A/1 -> [MPCC_f32Predictionterm_A]
  [MPCC_f32DGridVoltage] -> Product2/2
  Product1/1 -> Gain/1
  [MPCC_f32Predictionterm_C] -> Product1/1
  Product/1 -> Add1/1
  [MPCC_f32DVoltageVector2] -> Product4/2
  MPCC_f32DGridVoltage/1 -> [MPCC_f32DGridVoltage]
  [MPCC_f32Predictionterm_A] -> Product/1
  [MPCC_f32Predictionterm_B] -> Product4/1
  [MPCC_f32Predictionterm_B] -> Product2/1
  [MPCC_f32QGridCurrent_K_1] -> Product1/2
  MPCC_f32DGridCurrent_K_1/1 -> [MPCC_f32DGridCurrent_K_1]
  MPCC_f32QGridCurrent_K_1/1 -> [MPCC_f32QGridCurrent_K_1]
  MPCC_f32Predictionterm_C/1 -> [MPCC_f32Predictionterm_C]
  MPCC_f32Predictionterm_B/1 -> [MPCC_f32Predictionterm_B]
  Add1/1 -> MPCC_f32DGridCurrent_K_2_Voltage2/1
  MPCC_f32DVoltageVector2/1 -> [MPCC_f32DVoltageVector2]
  Product2/1 -> Add1/3
  Product4/1 -> Add1/4
  Gain/1 -> Add1/2

== system AB_Final_of_MPC_Bandwidth_Result_UnbalancedNew/Subsystem1/GridCurrentSecondPrediction/CostFunctionofVoltageVectors/CostFunctionVoltage2/QGridCurrentSecondPrediction_Voltage2 ==
  MPCC_f32Predictionterm_A : Inport
  MPCC_f32Predictionterm_B : Inport  Port=2
  MPCC_f32Predictionterm_C : Inport  Port=3
  MPCC_f32DGridCurrent_K_1 : Inport  Port=4
  MPCC_f32QGridCurrent_K_1 : Inport  Port=5
  MPCC_f32QGridVoltage : Inport  Port=6
  MPCC_f32QVoltageVector2 : Inport  Port=7
  Add1 : Sum  Inputs=+-+-
  Gain : Gain  Gain=0
  Product : Product
  Product1 : Product
  Product2 : Product  OutDataTypeStr=Inherit: Inherit via back propagation
  Product4 : Product
  MPCC_f32QGridCurrent_K_2_Voltage2 : Outport
  wires:
  [MPCC_f32QGridCurrent_K_1] -> Product/2
  MPCC_f32Predictionterm_A/1 -> [MPCC_f32Predictionterm_A]
  [MPCC_f32QGridVoltage] -> Product2/2
  Product1/1 -> Gain/1
  [MPCC_f32Predictionterm_C] -> Product1/1
  Product/1 -> Add1/1
  [MPCC_f32QVoltageVector2] -> Product4/2
  [MPCC_f32Predictionterm_A] -> Product/1
  [MPCC_f32Predictionterm_B] -> Product4/1
  [MPCC_f32Predictionterm_B] -> Product2/1
  [MPCC_f32DGridCurrent_K_1] -> Product1/2
  MPCC_f32DGridCurrent_K_1/1 -> [MPCC_f32DGridCurrent_K_1]
  MPCC_f32QGridCurrent_K_1/1 -> [MPCC_f32QGridCurrent_K_1]
  MPCC_f32Predictionterm_C/1 -> [MPCC_f32Predictionterm_C]
  MPCC_f32QGridVoltage/1 -> [MPCC_f32QGridVoltage]
  MPCC_f32Predictionterm_B/1 -> [MPCC_f32Predictionterm_B]
  Add1/1 -> MPCC_f32QGridCurrent_K_2_Voltage2/1
  MPCC_f32QVoltageVector2/1 -> [MPCC_f32QVoltageVector2]
  Product2/1 -> Add1/3
  Product4/1 -> Add1/4
  Gain/1 -> Add1/2

== system AB_Final_of_MPC_Bandwidth_Result_UnbalancedNew/Subsystem1/GridCurrentSecondPrediction/CostFunctionofVoltageVectors/CostFunctionVoltage3/CostFunctionVoltage3 ==
  MPCC_f32DGridCurrentReference : Inport
  MPCC_f32QGridCurrentReference : Inport  Port=2
  MPCC_f32DGridCurrent_K_2_Voltage3 : Inport  Port=3
  MPCC_f32QGridCurrent_K_2_Voltage3 : Inport  Port=4
  MPCC_f32DGridCurrent : Inport  Port=5
  MPCC_f32QGridCurrent : Inport  Port=6
  MPCC_f32DGridCurrent1 : Inport  Port=7
  MPCC_f32QGridCurrent1 : Inport  Port=8
  Abs{,1..5} (6 alike) : Abs  SaturateOnIntegerOverflow=off
  Add{,2..6} (6 alike) : Sum  Inputs=+-
  Add1 : Sum  Inputs=++++++
  Constant : Constant  Value=single(0)
  Constant1 : Constant  Value=single(0)
  Gain : Gain
  Gain1 : Gain
  Gain2 : Gain  Gain=0
  Gain3 : Gain  Gain=0
  Square : Math  Operator=square
  Square1 : Math  Operator=square
  MPCC_f32CostFunction_Voltage3 : Outport
  wires:
  MPCC_f32QGridCurrentReference/1 -> [MPCC_f32QGridCurrentReference]
  MPCC_f32DGridCurrentReference/1 -> [MPCC_f32DGridCurrentReference]
  MPCC_f32QGridCurrent_K_2_Voltage3/1 -> [MPCC_f32QGridCurrent_K_2_Voltage3]
  MPCC_f32DGridCurrent_K_2_Voltage3/1 -> [MPCC_f32DGridCurrent_K_2_Voltage3]
  [MPCC_f32DGridCurrentReference] -> Add/1
  [MPCC_f32DGridCurrent_K_2_Voltage3] -> Add/2
  [MPCC_f32QGridCurrentReference] -> Add2/1
  [MPCC_f32QGridCurrent_K_2_Voltage3] -> Add2/2
  MPCC_f32QGridCurrent/1 -> [MPCC_f32QGridCurrent]
  MPCC_f32DGridCurrent/1 -> [MPCC_f32DGridCurrent]
  [MPCC_f32QGridCurrent] -> Add4/1
  Add4/1 -> Abs3/1
  Add3/1 -> Abs2/1
  [MPCC_f32QGridCurrent_K_2_Voltage3] -> Add4/2
  [MPCC_f32DGridCurrent] -> Add3/1
  [MPCC_f32DGridCurrent_K_2_Voltage3] -> Add3/2
  Abs2/1 -> Gain/1
  Abs3/1 -> Gain1/1
  Add1/1 -> MPCC_f32CostFunction_Voltage3/1
  Gain/1 -> Add1/3
  Gain1/1 -> Add1/4
  Abs1/1 -> Add1/2
  Add2/1 -> Abs1/1
  Abs/1 -> Add1/1
  Add/1 -> Abs/1
  MPCC_f32DGridCurrent1/1 -> [MPCC_f32DGridCurrent1]
  MPCC_f32QGridCurrent1/1 -> [MPCC_f32QGridCurrent1]
  Constant/1 -> Add5/1
  Add5/1 -> Abs4/1
  Add6/1 -> Abs5/1
  Abs4/1 -> Gain2/1
  Constant1/1 -> Add6/1
  [MPCC_f32DGridCurrent1] -> Add6/2
  [MPCC_f32QGridCurrent1] -> Add5/2
  Gain2/1 -> Add1/6
  Abs5/1 -> Gain3/1
  Gain3/1 -> Add1/5

== system AB_Final_of_MPC_Bandwidth_Result_UnbalancedNew/Subsystem1/GridCurrentSecondPrediction/CostFunctionofVoltageVectors/CostFunctionVoltage3/DGridCurrentSecondPrediction_Voltage3 ==
  MPCC_f32Predictionterm_A : Inport
  MPCC_f32Predictionterm_B : Inport  Port=2
  MPCC_f32Predictionterm_C : Inport  Port=3
  MPCC_f32DGridCurrent_K_1 : Inport  Port=4
  MPCC_f32QGridCurrent_K_1 : Inport  Port=5
  MPCC_f32DGridVoltage : Inport  Port=6
  MPCC_f32DVoltageVector3 : Inport  Port=7
  Add1 : Sum  Inputs=+++-
  Gain : Gain  Gain=0
  Product : Product
  Product1 : Product
  Product2 : Product  OutDataTypeStr=Inherit: Inherit via back propagation
  Product4 : Product
  MPCC_f32DGridCurrent_K_2_Voltage3 : Outport
  wires:
  [MPCC_f32DGridCurrent_K_1] -> Product/2
  MPCC_f32Predictionterm_A/1 -> [MPCC_f32Predictionterm_A]
  [MPCC_f32DGridVoltage] -> Product2/2
  Product1/1 -> Gain/1
  [MPCC_f32Predictionterm_C] -> Product1/1
  Product/1 -> Add1/1
  [MPCC_f32DVoltageVector3] -> Product4/2
  MPCC_f32DGridVoltage/1 -> [MPCC_f32DGridVoltage]
  [MPCC_f32Predictionterm_A] -> Product/1
  [MPCC_f32Predictionterm_B] -> Product4/1
  [MPCC_f32Predictionterm_B] -> Product2/1
  [MPCC_f32QGridCurrent_K_1] -> Product1/2
  MPCC_f32DGridCurrent_K_1/1 -> [MPCC_f32DGridCurrent_K_1]
  MPCC_f32QGridCurrent_K_1/1 -> [MPCC_f32QGridCurrent_K_1]
  MPCC_f32Predictionterm_C/1 -> [MPCC_f32Predictionterm_C]
  MPCC_f32Predictionterm_B/1 -> [MPCC_f32Predictionterm_B]
  Add1/1 -> MPCC_f32DGridCurrent_K_2_Voltage3/1
  MPCC_f32DVoltageVector3/1 -> [MPCC_f32DVoltageVector3]
  Product2/1 -> Add1/3
  Product4/1 -> Add1/4
  Gain/1 -> Add1/2

== system AB_Final_of_MPC_Bandwidth_Result_UnbalancedNew/Subsystem1/GridCurrentSecondPrediction/CostFunctionofVoltageVectors/CostFunctionVoltage3/QGridCurrentSecondPrediction_Voltage3 ==
  MPCC_f32Predictionterm_A : Inport
  MPCC_f32Predictionterm_B : Inport  Port=2
  MPCC_f32Predictionterm_C : Inport  Port=3
  MPCC_f32DGridCurrent_K_1 : Inport  Port=4
  MPCC_f32QGridCurrent_K_1 : Inport  Port=5
  MPCC_f32QGridVoltage : Inport  Port=6
  MPCC_f32QVoltageVector3 : Inport  Port=7
  Add1 : Sum  Inputs=+-+-
  Gain : Gain  Gain=0
  Product : Product
  Product1 : Product
  Product2 : Product  OutDataTypeStr=Inherit: Inherit via back propagation
  Product4 : Product
  MPCC_f32QGridCurrent_K_2_Voltage3 : Outport
  wires:
  [MPCC_f32QGridCurrent_K_1] -> Product/2
  MPCC_f32Predictionterm_A/1 -> [MPCC_f32Predictionterm_A]
  [MPCC_f32QGridVoltage] -> Product2/2
  Product1/1 -> Gain/1
  [MPCC_f32Predictionterm_C] -> Product1/1
  Product/1 -> Add1/1
  [MPCC_f32QVoltageVector3] -> Product4/2
  [MPCC_f32Predictionterm_A] -> Product/1
  [MPCC_f32Predictionterm_B] -> Product4/1
  [MPCC_f32Predictionterm_B] -> Product2/1
  [MPCC_f32DGridCurrent_K_1] -> Product1/2
  MPCC_f32DGridCurrent_K_1/1 -> [MPCC_f32DGridCurrent_K_1]
  MPCC_f32QGridCurrent_K_1/1 -> [MPCC_f32QGridCurrent_K_1]
  MPCC_f32Predictionterm_C/1 -> [MPCC_f32Predictionterm_C]
  MPCC_f32QGridVoltage/1 -> [MPCC_f32QGridVoltage]
  MPCC_f32Predictionterm_B/1 -> [MPCC_f32Predictionterm_B]
  Add1/1 -> MPCC_f32QGridCurrent_K_2_Voltage3/1
  MPCC_f32QVoltageVector3/1 -> [MPCC_f32QVoltageVector3]
  Product2/1 -> Add1/3
  Product4/1 -> Add1/4
  Gain/1 -> Add1/2

== system AB_Final_of_MPC_Bandwidth_Result_UnbalancedNew/Subsystem1/GridCurrentSecondPrediction/CostFunctionofVoltageVectors/CostFunctionVoltage4/CostFunctionVoltage4 ==
  MPCC_f32DGridCurrentReference : Inport
  MPCC_f32QGridCurrentReference : Inport  Port=2
  MPCC_f32DGridCurrent_K_2_Voltage4 : Inport  Port=3
  MPCC_f32QGridCurrent_K_2_Voltage4 : Inport  Port=4
  MPCC_f32DGridCurrent : Inport  Port=5
  MPCC_f32QGridCurrent : Inport  Port=6
  MPCC_f32DGridCurrent1 : Inport  Port=7
  MPCC_f32QGridCurrent1 : Inport  Port=8
  Abs{,1..5} (6 alike) : Abs  SaturateOnIntegerOverflow=off
  Add{,2..6} (6 alike) : Sum  Inputs=+-
  Add1 : Sum  Inputs=++++++
  Constant : Constant  Value=single(0)
  Constant1 : Constant  Value=single(0)
  Gain : Gain
  Gain1 : Gain
  Gain2 : Gain  Gain=0
  Gain3 : Gain  Gain=0
  Square : Math  Operator=square
  Square1 : Math  Operator=square
  MPCC_f32CostFunction_Voltage4 : Outport
  wires:
  MPCC_f32QGridCurrentReference/1 -> [MPCC_f32QGridCurrentReference]
  MPCC_f32DGridCurrentReference/1 -> [MPCC_f32DGridCurrentReference]
  MPCC_f32QGridCurrent_K_2_Voltage4/1 -> [MPCC_f32QGridCurrent_K_2_Voltage4]
  MPCC_f32DGridCurrent_K_2_Voltage4/1 -> [MPCC_f32DGridCurrent_K_2_Voltage4]
  [MPCC_f32DGridCurrentReference] -> Add/1
  [MPCC_f32DGridCurrent_K_2_Voltage4] -> Add/2
  [MPCC_f32QGridCurrentReference] -> Add2/1
  [MPCC_f32QGridCurrent_K_2_Voltage4] -> Add2/2
  MPCC_f32QGridCurrent/1 -> [MPCC_f32QGridCurrent]
  MPCC_f32DGridCurrent/1 -> [MPCC_f32DGridCurrent]
  [MPCC_f32QGridCurrent] -> Add4/1
  Add4/1 -> Abs3/1
  Add3/1 -> Abs2/1
  [MPCC_f32QGridCurrent_K_2_Voltage4] -> Add4/2
  [MPCC_f32DGridCurrent] -> Add3/1
  [MPCC_f32DGridCurrent_K_2_Voltage4] -> Add3/2
  Abs2/1 -> Gain/1
  Abs3/1 -> Gain1/1
  Add1/1 -> MPCC_f32CostFunction_Voltage4/1
  Gain/1 -> Add1/3
  Gain1/1 -> Add1/4
  Abs1/1 -> Add1/2
  Add2/1 -> Abs1/1
  Abs/1 -> Add1/1
  Add/1 -> Abs/1
  MPCC_f32DGridCurrent1/1 -> [MPCC_f32DGridCurrent1]
  MPCC_f32QGridCurrent1/1 -> [MPCC_f32QGridCurrent1]
  Constant/1 -> Add5/1
  Add5/1 -> Abs4/1
  Add6/1 -> Abs5/1
  Abs4/1 -> Gain2/1
  Constant1/1 -> Add6/1
  [MPCC_f32DGridCurrent1] -> Add6/2
  [MPCC_f32QGridCurrent1] -> Add5/2
  Gain2/1 -> Add1/6
  Abs5/1 -> Gain3/1
  Gain3/1 -> Add1/5
